simulink subsystem "get_edge_squared"  (R2025b)
settings: Solver=VariableStepAuto  StartTime=0.0  StopTime=10.0  RelTol=1e-3
settings Model: Creator=adam  LastModifiedBy=aherrman

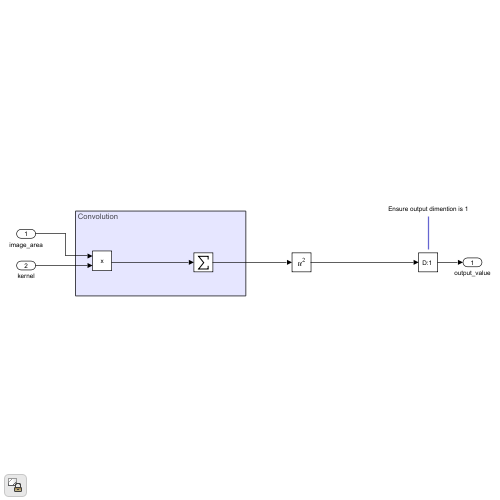
[thumbnail: Simulink's stored preview of the top-level diagram]
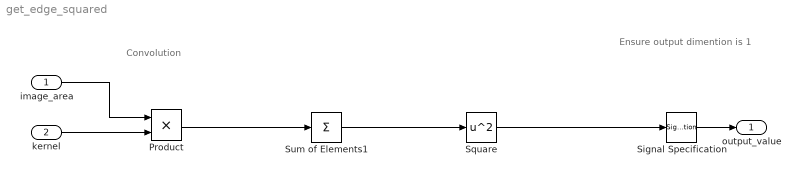
== system get_edge_squared ==
  note: Ensure output dimention is 1
  note: Convolution
  image_area : Inport
  kernel : Inport  Port=2
  Product : Product
  Signal Specification : SignalSpecification  Dimensions=1
  Square : Math  Operator=square
  Sum of Elements1 : Sum  Inputs=+
  output_value : Outport
  wires:
  Sum of Elements1/1 -> Square/1
  Signal Specification/1 -> output_value/1
  Product/1 -> Sum of Elements1/1
  Square/1 -> Signal Specification/1
  kernel/1 -> Product/2
  image_area/1 -> Product/1
